simulink model "generic_src"  (Simulink 10.3)
settings: Solver=ode45  StartTime=0.0  StopTime=inf  RelTol=1e-3  EnableMultiTasking=on
undefined symbols (not defined in the file): Area_Front, Area_Rear, ay_max_off, ay_max_on, ay_per_mu_max_off, ay_per_mu_max_on, Brake_ratio, brake_valve_ctrl_kP, cat1mode1_higher, cat1mode1_lower, cat1mode2_higher, cat1mode2_lower, cat1mode3_higher, cat1mode3_lower, cat2mode1_higher, cat2mode1_lower, cat2mode2_higher, cat2mode2_lower, cat2mode3_higher, cat2mode3_lower, delta_vel, diff_lock_fac, diff_lock_off, diff_lock_on, ESP_ctrl_kD, ESP_ctrl_kI, ESP_ctrl_kP, ESP_ctrl_restore_kI, ESP_min_throttle_fac, f_ax, f_slip, g, higherlimit_highvel, higherlimit_lowvel, highervel_fac, highervelocity_fac, InitialConditionForIntegrator, limit_acc, limit_selectlow, limit_starting, limit_vdiff, locktime_throttle, lowerlimit_highvel, lowerlimit_lowvel, lowervel_fac, lowervelocity_fac, min_throttle, MPS2KMPH, MSR_ctrl_kD, MSR_ctrl_kI, MSR_ctrl_kP, MSR_min_throttle_fac, PID_kP_sideslip, PID_kP_yawrate, RADpS2RpM, rBrake, RpM2RADpS, SH_SL_switch, sideslip_vel_corr, sidesplip_deviation_max ... (+35)
libraries: CarMaker4SL x137, simulink x57, simulink_extras x6
(part 5 of 12)

== system generic_src/CarMaker/IPG Vehicle/PowerTrain/PTControl Example/PTC ClutchOut/CreateBus PTC ClutchOut2 ==
  In : Inport
  BusCreator : BusCreator  Inputs=3
  Demux : Demux  Outputs=3
      settings: DisplayOption=none
  Out : Outport  VectorParamsAs1DForOutWhenUnconnected=off
  wires:
  Demux/3 -> BusCreator/3  "PTC ClutchOut2 Trq_out_trg"
  Demux/2 -> BusCreator/2  "PTC ClutchOut2 rotv_out_trg"
  Demux/1 -> BusCreator/1  "PTC ClutchOut2 Pos"
  BusCreator/1 -> Out/1
  In/1 -> Demux/1

== system generic_src/CarMaker/IPG Vehicle/PowerTrain/PTControl Example/PTC ClutchOut/CreateBus PTC ClutchOut3 ==
  In : Inport
  BusCreator : BusCreator  Inputs=3
  Demux : Demux  Outputs=3
      settings: DisplayOption=none
  Out : Outport  VectorParamsAs1DForOutWhenUnconnected=off
  wires:
  Demux/3 -> BusCreator/3  "PTC ClutchOut3 Trq_out_trg"
  Demux/2 -> BusCreator/2  "PTC ClutchOut3 rotv_out_trg"
  Demux/1 -> BusCreator/1  "PTC ClutchOut3 Pos"
  BusCreator/1 -> Out/1
  In/1 -> Demux/1

== system generic_src/CarMaker/IPG Vehicle/PowerTrain/PTControl Example/PTC ClutchOut/CreateBus PTC ClutchOut4 ==
  In : Inport
  BusCreator : BusCreator  Inputs=3
  Demux : Demux  Outputs=3
      settings: DisplayOption=none
  Out : Outport  VectorParamsAs1DForOutWhenUnconnected=off
  wires:
  Demux/3 -> BusCreator/3  "PTC ClutchOut4 Trq_out_trg"
  Demux/2 -> BusCreator/2  "PTC ClutchOut4 rotv_out_trg"
  Demux/1 -> BusCreator/1  "PTC ClutchOut4 Pos"
  BusCreator/1 -> Out/1
  In/1 -> Demux/1

== system generic_src/CarMaker/IPG Vehicle/PowerTrain/PTControl Example/PTC ClutchOut/CreateBus PTC ClutchOut5 ==
  In : Inport
  BusCreator : BusCreator  Inputs=3
  Demux : Demux  Outputs=3
      settings: DisplayOption=none
  Out : Outport  VectorParamsAs1DForOutWhenUnconnected=off
  wires:
  Demux/3 -> BusCreator/3  "PTC ClutchOut5 Trq_out_trg"
  Demux/2 -> BusCreator/2  "PTC ClutchOut5 rotv_out_trg"
  Demux/1 -> BusCreator/1  "PTC ClutchOut5 Pos"
  BusCreator/1 -> Out/1
  In/1 -> Demux/1

== system generic_src/CarMaker/IPG Vehicle/PowerTrain/PTControl Example/PTC ClutchOut/CreateBus PTC ClutchOut6 ==
  In : Inport
  BusCreator : BusCreator  Inputs=3
  Demux : Demux  Outputs=3
      settings: DisplayOption=none
  Out : Outport  VectorParamsAs1DForOutWhenUnconnected=off
  wires:
  Demux/3 -> BusCreator/3  "PTC ClutchOut6 Trq_out_trg"
  Demux/2 -> BusCreator/2  "PTC ClutchOut6 rotv_out_trg"
  Demux/1 -> BusCreator/1  "PTC ClutchOut6 Pos"
  BusCreator/1 -> Out/1
  In/1 -> Demux/1

== system generic_src/CarMaker/IPG Vehicle/PowerTrain/PTControl Example/PTC ClutchOut/CreateBus PTC ClutchOut7 ==
  In : Inport
  BusCreator : BusCreator  Inputs=3
  Demux : Demux  Outputs=3
      settings: DisplayOption=none
  Out : Outport  VectorParamsAs1DForOutWhenUnconnected=off
  wires:
  Demux/3 -> BusCreator/3  "PTC ClutchOut7 Trq_out_trg"
  Demux/2 -> BusCreator/2  "PTC ClutchOut7 rotv_out_trg"
  Demux/1 -> BusCreator/1  "PTC ClutchOut7 Pos"
  BusCreator/1 -> Out/1
  In/1 -> Demux/1

== system generic_src/CarMaker/IPG Vehicle/PowerTrain/PTControl Example/PTC ClutchOut/CreateBus PTC ClutchOut8 ==
  In : Inport
  BusCreator : BusCreator  Inputs=3
  Demux : Demux  Outputs=3
      settings: DisplayOption=none
  Out : Outport  VectorParamsAs1DForOutWhenUnconnected=off
  wires:
  Demux/3 -> BusCreator/3  "PTC ClutchOut8 Trq_out_trg"
  Demux/2 -> BusCreator/2  "PTC ClutchOut8 rotv_out_trg"
  Demux/1 -> BusCreator/1  "PTC ClutchOut8 Pos"
  BusCreator/1 -> Out/1
  In/1 -> Demux/1

== system generic_src/CarMaker/IPG Vehicle/PowerTrain/PTControl Example/PTC ClutchOut/CreateBus PTC ClutchOut9 ==
  In : Inport
  BusCreator : BusCreator  Inputs=3
  Demux : Demux  Outputs=3
      settings: DisplayOption=none
  Out : Outport  VectorParamsAs1DForOutWhenUnconnected=off
  wires:
  Demux/3 -> BusCreator/3  "PTC ClutchOut9 Trq_out_trg"
  Demux/2 -> BusCreator/2  "PTC ClutchOut9 rotv_out_trg"
  Demux/1 -> BusCreator/1  "PTC ClutchOut9 Pos"
  BusCreator/1 -> Out/1
  In/1 -> Demux/1

== system generic_src/CarMaker/IPG Vehicle/PowerTrain/PTControl Example/PTC GearBoxOut/CreateBus PTC GearboxOut0 ==
  In : Inport
  BusCreator : BusCreator  Inputs=12
  Demux : Demux  Outputs=12
      settings: DisplayOption=none
  Out : Outport  VectorParamsAs1DForOutWhenUnconnected=off
  wires:
  Demux/12 -> BusCreator/12  "PTC GearboxOut0 Clutch_dis Trq_out_trg"
  Demux/11 -> BusCreator/11  "PTC GearboxOut0 Clutch_dis rotv_out_trg"
  Demux/10 -> BusCreator/10  "PTC GearboxOut0 Clutch_dis Pos"
  Demux/9 -> BusCreator/9  "PTC GearboxOut0 Clutch Trq_out_trg"
  Demux/8 -> BusCreator/8  "PTC GearboxOut0 Clutch rotv_out_trg"
  Demux/7 -> BusCreator/7  "PTC GearboxOut0 Clutch Pos"
  Demux/6 -> BusCreator/6  "PTC GearboxOut0 Trq_out_trg"
  Demux/5 -> BusCreator/5  "PTC GearboxOut0 rotv_in_trg"
  Demux/4 -> BusCreator/4  "PTC GearboxOut0 i_trg"
  Demux/3 -> BusCreator/3  "PTC GearboxOut0 set_ParkBrake"
  Demux/2 -> BusCreator/2  "PTC GearboxOut0 GearNoTrg_dis"
  Demux/1 -> BusCreator/1  "PTC GearboxOut0 GearNoTrg"
  BusCreator/1 -> Out/1
  In/1 -> Demux/1

== system generic_src/CarMaker/IPG Vehicle/PowerTrain/PTControl Example/PTC GearBoxOut/CreateBus PTC GearboxOut1 ==
  In : Inport
  BusCreator : BusCreator  Inputs=12
  Demux : Demux  Outputs=12
      settings: DisplayOption=none
  Out : Outport  VectorParamsAs1DForOutWhenUnconnected=off
  wires:
  Demux/12 -> BusCreator/12  "PTC GearboxOut1 Clutch_dis Trq_out_trg"
  Demux/11 -> BusCreator/11  "PTC GearboxOut1 Clutch_dis rotv_out_trg"
  Demux/10 -> BusCreator/10  "PTC GearboxOut1 Clutch_dis Pos"
  Demux/9 -> BusCreator/9  "PTC GearboxOut1 Clutch Trq_out_trg"
  Demux/8 -> BusCreator/8  "PTC GearboxOut1 Clutch rotv_out_trg"
  Demux/7 -> BusCreator/7  "PTC GearboxOut1 Clutch Pos"
  Demux/6 -> BusCreator/6  "PTC GearboxOut1 Trq_out_trg"
  Demux/5 -> BusCreator/5  "PTC GearboxOut1 rotv_in_trg"
  Demux/4 -> BusCreator/4  "PTC GearboxOut1 i_trg"
  Demux/3 -> BusCreator/3  "PTC GearboxOut1 set_ParkBrake"
  Demux/2 -> BusCreator/2  "PTC GearboxOut1 GearNoTrg_dis"
  Demux/1 -> BusCreator/1  "PTC GearboxOut1 GearNoTrg"
  BusCreator/1 -> Out/1
  In/1 -> Demux/1

== system generic_src/CarMaker/IPG Vehicle/PowerTrain/PTControl Example/PTC GearBoxOut/CreateBus PTC GearboxOut10 ==
  In : Inport
  BusCreator : BusCreator  Inputs=12
  Demux : Demux  Outputs=12
      settings: DisplayOption=none
  Out : Outport  VectorParamsAs1DForOutWhenUnconnected=off
  wires:
  Demux/12 -> BusCreator/12  "PTC GearboxOut10 Clutch_dis Trq_out_trg"
  Demux/11 -> BusCreator/11  "PTC GearboxOut10 Clutch_dis rotv_out_trg"
  Demux/10 -> BusCreator/10  "PTC GearboxOut10 Clutch_dis Pos"
  Demux/9 -> BusCreator/9  "PTC GearboxOut10 Clutch Trq_out_trg"
  Demux/8 -> BusCreator/8  "PTC GearboxOut10 Clutch rotv_out_trg"
  Demux/7 -> BusCreator/7  "PTC GearboxOut10 Clutch Pos"
  Demux/6 -> BusCreator/6  "PTC GearboxOut10 Trq_out_trg"
  Demux/5 -> BusCreator/5  "PTC GearboxOut10 rotv_in_trg"
  Demux/4 -> BusCreator/4  "PTC GearboxOut10 i_trg"
  Demux/3 -> BusCreator/3  "PTC GearboxOut10 set_ParkBrake"
  Demux/2 -> BusCreator/2  "PTC GearboxOut10 GearNoTrg_dis"
  Demux/1 -> BusCreator/1  "PTC GearboxOut10 GearNoTrg"
  BusCreator/1 -> Out/1
  In/1 -> Demux/1

== system generic_src/CarMaker/IPG Vehicle/PowerTrain/PTControl Example/PTC GearBoxOut/CreateBus PTC GearboxOut11 ==
  In : Inport
  BusCreator : BusCreator  Inputs=12
  Demux : Demux  Outputs=12
      settings: DisplayOption=none
  Out : Outport  VectorParamsAs1DForOutWhenUnconnected=off
  wires:
  Demux/12 -> BusCreator/12  "PTC GearboxOut11 Clutch_dis Trq_out_trg"
  Demux/11 -> BusCreator/11  "PTC GearboxOut11 Clutch_dis rotv_out_trg"
  Demux/10 -> BusCreator/10  "PTC GearboxOut11 Clutch_dis Pos"
  Demux/9 -> BusCreator/9  "PTC GearboxOut11 Clutch Trq_out_trg"
  Demux/8 -> BusCreator/8  "PTC GearboxOut11 Clutch rotv_out_trg"
  Demux/7 -> BusCreator/7  "PTC GearboxOut11 Clutch Pos"
  Demux/6 -> BusCreator/6  "PTC GearboxOut11 Trq_out_trg"
  Demux/5 -> BusCreator/5  "PTC GearboxOut11 rotv_in_trg"
  Demux/4 -> BusCreator/4  "PTC GearboxOut11 i_trg"
  Demux/3 -> BusCreator/3  "PTC GearboxOut11 set_ParkBrake"
  Demux/2 -> BusCreator/2  "PTC GearboxOut11 GearNoTrg_dis"
  Demux/1 -> BusCreator/1  "PTC GearboxOut11 GearNoTrg"
  BusCreator/1 -> Out/1
  In/1 -> Demux/1

== system generic_src/CarMaker/IPG Vehicle/PowerTrain/PTControl Example/PTC GearBoxOut/CreateBus PTC GearboxOut2 ==
  In : Inport
  BusCreator : BusCreator  Inputs=12
  Demux : Demux  Outputs=12
      settings: DisplayOption=none
  Out : Outport  VectorParamsAs1DForOutWhenUnconnected=off
  wires:
  Demux/12 -> BusCreator/12  "PTC GearboxOut2 Clutch_dis Trq_out_trg"
  Demux/11 -> BusCreator/11  "PTC GearboxOut2 Clutch_dis rotv_out_trg"
  Demux/10 -> BusCreator/10  "PTC GearboxOut2 Clutch_dis Pos"
  Demux/9 -> BusCreator/9  "PTC GearboxOut2 Clutch Trq_out_trg"
  Demux/8 -> BusCreator/8  "PTC GearboxOut2 Clutch rotv_out_trg"
  Demux/7 -> BusCreator/7  "PTC GearboxOut2 Clutch Pos"
  Demux/6 -> BusCreator/6  "PTC GearboxOut2 Trq_out_trg"
  Demux/5 -> BusCreator/5  "PTC GearboxOut2 rotv_in_trg"
  Demux/4 -> BusCreator/4  "PTC GearboxOut2 i_trg"
  Demux/3 -> BusCreator/3  "PTC GearboxOut2 set_ParkBrake"
  Demux/2 -> BusCreator/2  "PTC GearboxOut2 GearNoTrg_dis"
  Demux/1 -> BusCreator/1  "PTC GearboxOut2 GearNoTrg"
  BusCreator/1 -> Out/1
  In/1 -> Demux/1

== system generic_src/CarMaker/IPG Vehicle/PowerTrain/PTControl Example/PTC GearBoxOut/CreateBus PTC GearboxOut3 ==
  In : Inport
  BusCreator : BusCreator  Inputs=12
  Demux : Demux  Outputs=12
      settings: DisplayOption=none
  Out : Outport  VectorParamsAs1DForOutWhenUnconnected=off
  wires:
  Demux/12 -> BusCreator/12  "PTC GearboxOut3 Clutch_dis Trq_out_trg"
  Demux/11 -> BusCreator/11  "PTC GearboxOut3 Clutch_dis rotv_out_trg"
  Demux/10 -> BusCreator/10  "PTC GearboxOut3 Clutch_dis Pos"
  Demux/9 -> BusCreator/9  "PTC GearboxOut3 Clutch Trq_out_trg"
  Demux/8 -> BusCreator/8  "PTC GearboxOut3 Clutch rotv_out_trg"
  Demux/7 -> BusCreator/7  "PTC GearboxOut3 Clutch Pos"
  Demux/6 -> BusCreator/6  "PTC GearboxOut3 Trq_out_trg"
  Demux/5 -> BusCreator/5  "PTC GearboxOut3 rotv_in_trg"
  Demux/4 -> BusCreator/4  "PTC GearboxOut3 i_trg"
  Demux/3 -> BusCreator/3  "PTC GearboxOut3 set_ParkBrake"
  Demux/2 -> BusCreator/2  "PTC GearboxOut3 GearNoTrg_dis"
  Demux/1 -> BusCreator/1  "PTC GearboxOut3 GearNoTrg"
  BusCreator/1 -> Out/1
  In/1 -> Demux/1

== system generic_src/CarMaker/IPG Vehicle/PowerTrain/PTControl Example/PTC GearBoxOut/CreateBus PTC GearboxOut4 ==
  In : Inport
  BusCreator : BusCreator  Inputs=12
  Demux : Demux  Outputs=12
      settings: DisplayOption=none
  Out : Outport  VectorParamsAs1DForOutWhenUnconnected=off
  wires:
  Demux/12 -> BusCreator/12  "PTC GearboxOut4 Clutch_dis Trq_out_trg"
  Demux/11 -> BusCreator/11  "PTC GearboxOut4 Clutch_dis rotv_out_trg"
  Demux/10 -> BusCreator/10  "PTC GearboxOut4 Clutch_dis Pos"
  Demux/9 -> BusCreator/9  "PTC GearboxOut4 Clutch Trq_out_trg"
  Demux/8 -> BusCreator/8  "PTC GearboxOut4 Clutch rotv_out_trg"
  Demux/7 -> BusCreator/7  "PTC GearboxOut4 Clutch Pos"
  Demux/6 -> BusCreator/6  "PTC GearboxOut4 Trq_out_trg"
  Demux/5 -> BusCreator/5  "PTC GearboxOut4 rotv_in_trg"
  Demux/4 -> BusCreator/4  "PTC GearboxOut4 i_trg"
  Demux/3 -> BusCreator/3  "PTC GearboxOut4 set_ParkBrake"
  Demux/2 -> BusCreator/2  "PTC GearboxOut4 GearNoTrg_dis"
  Demux/1 -> BusCreator/1  "PTC GearboxOut4 GearNoTrg"
  BusCreator/1 -> Out/1
  In/1 -> Demux/1

== system generic_src/CarMaker/IPG Vehicle/PowerTrain/PTControl Example/PTC GearBoxOut/CreateBus PTC GearboxOut5 ==
  In : Inport
  BusCreator : BusCreator  Inputs=12
  Demux : Demux  Outputs=12
      settings: DisplayOption=none
  Out : Outport  VectorParamsAs1DForOutWhenUnconnected=off
  wires:
  Demux/12 -> BusCreator/12  "PTC GearboxOut5 Clutch_dis Trq_out_trg"
  Demux/11 -> BusCreator/11  "PTC GearboxOut5 Clutch_dis rotv_out_trg"
  Demux/10 -> BusCreator/10  "PTC GearboxOut5 Clutch_dis Pos"
  Demux/9 -> BusCreator/9  "PTC GearboxOut5 Clutch Trq_out_trg"
  Demux/8 -> BusCreator/8  "PTC GearboxOut5 Clutch rotv_out_trg"
  Demux/7 -> BusCreator/7  "PTC GearboxOut5 Clutch Pos"
  Demux/6 -> BusCreator/6  "PTC GearboxOut5 Trq_out_trg"
  Demux/5 -> BusCreator/5  "PTC GearboxOut5 rotv_in_trg"
  Demux/4 -> BusCreator/4  "PTC GearboxOut5 i_trg"
  Demux/3 -> BusCreator/3  "PTC GearboxOut5 set_ParkBrake"
  Demux/2 -> BusCreator/2  "PTC GearboxOut5 GearNoTrg_dis"
  Demux/1 -> BusCreator/1  "PTC GearboxOut5 GearNoTrg"
  BusCreator/1 -> Out/1
  In/1 -> Demux/1

== system generic_src/CarMaker/IPG Vehicle/PowerTrain/PTControl Example/PTC GearBoxOut/CreateBus PTC GearboxOut6 ==
  In : Inport
  BusCreator : BusCreator  Inputs=12
  Demux : Demux  Outputs=12
      settings: DisplayOption=none
  Out : Outport  VectorParamsAs1DForOutWhenUnconnected=off
  wires:
  Demux/12 -> BusCreator/12  "PTC GearboxOut6 Clutch_dis Trq_out_trg"
  Demux/11 -> BusCreator/11  "PTC GearboxOut6 Clutch_dis rotv_out_trg"
  Demux/10 -> BusCreator/10  "PTC GearboxOut6 Clutch_dis Pos"
  Demux/9 -> BusCreator/9  "PTC GearboxOut6 Clutch Trq_out_trg"
  Demux/8 -> BusCreator/8  "PTC GearboxOut6 Clutch rotv_out_trg"
  Demux/7 -> BusCreator/7  "PTC GearboxOut6 Clutch Pos"
  Demux/6 -> BusCreator/6  "PTC GearboxOut6 Trq_out_trg"
  Demux/5 -> BusCreator/5  "PTC GearboxOut6 rotv_in_trg"
  Demux/4 -> BusCreator/4  "PTC GearboxOut6 i_trg"
  Demux/3 -> BusCreator/3  "PTC GearboxOut6 set_ParkBrake"
  Demux/2 -> BusCreator/2  "PTC GearboxOut6 GearNoTrg_dis"
  Demux/1 -> BusCreator/1  "PTC GearboxOut6 GearNoTrg"
  BusCreator/1 -> Out/1
  In/1 -> Demux/1

== system generic_src/CarMaker/IPG Vehicle/PowerTrain/PTControl Example/PTC GearBoxOut/CreateBus PTC GearboxOut7 ==
  In : Inport
  BusCreator : BusCreator  Inputs=12
  Demux : Demux  Outputs=12
      settings: DisplayOption=none
  Out : Outport  VectorParamsAs1DForOutWhenUnconnected=off
  wires:
  Demux/12 -> BusCreator/12  "PTC GearboxOut7 Clutch_dis Trq_out_trg"
  Demux/11 -> BusCreator/11  "PTC GearboxOut7 Clutch_dis rotv_out_trg"
  Demux/10 -> BusCreator/10  "PTC GearboxOut7 Clutch_dis Pos"
  Demux/9 -> BusCreator/9  "PTC GearboxOut7 Clutch Trq_out_trg"
  Demux/8 -> BusCreator/8  "PTC GearboxOut7 Clutch rotv_out_trg"
  Demux/7 -> BusCreator/7  "PTC GearboxOut7 Clutch Pos"
  Demux/6 -> BusCreator/6  "PTC GearboxOut7 Trq_out_trg"
  Demux/5 -> BusCreator/5  "PTC GearboxOut7 rotv_in_trg"
  Demux/4 -> BusCreator/4  "PTC GearboxOut7 i_trg"
  Demux/3 -> BusCreator/3  "PTC GearboxOut7 set_ParkBrake"
  Demux/2 -> BusCreator/2  "PTC GearboxOut7 GearNoTrg_dis"
  Demux/1 -> BusCreator/1  "PTC GearboxOut7 GearNoTrg"
  BusCreator/1 -> Out/1
  In/1 -> Demux/1

== system generic_src/CarMaker/IPG Vehicle/PowerTrain/PTControl Example/PTC GearBoxOut/CreateBus PTC GearboxOut8 ==
  In : Inport
  BusCreator : BusCreator  Inputs=12
  Demux : Demux  Outputs=12
      settings: DisplayOption=none
  Out : Outport  VectorParamsAs1DForOutWhenUnconnected=off
  wires:
  Demux/12 -> BusCreator/12  "PTC GearboxOut8 Clutch_dis Trq_out_trg"
  Demux/11 -> BusCreator/11  "PTC GearboxOut8 Clutch_dis rotv_out_trg"
  Demux/10 -> BusCreator/10  "PTC GearboxOut8 Clutch_dis Pos"
  Demux/9 -> BusCreator/9  "PTC GearboxOut8 Clutch Trq_out_trg"
  Demux/8 -> BusCreator/8  "PTC GearboxOut8 Clutch rotv_out_trg"
  Demux/7 -> BusCreator/7  "PTC GearboxOut8 Clutch Pos"
  Demux/6 -> BusCreator/6  "PTC GearboxOut8 Trq_out_trg"
  Demux/5 -> BusCreator/5  "PTC GearboxOut8 rotv_in_trg"
  Demux/4 -> BusCreator/4  "PTC GearboxOut8 i_trg"
  Demux/3 -> BusCreator/3  "PTC GearboxOut8 set_ParkBrake"
  Demux/2 -> BusCreator/2  "PTC GearboxOut8 GearNoTrg_dis"
  Demux/1 -> BusCreator/1  "PTC GearboxOut8 GearNoTrg"
  BusCreator/1 -> Out/1
  In/1 -> Demux/1

== system generic_src/CarMaker/IPG Vehicle/PowerTrain/PTControl Example/PTC GearBoxOut/CreateBus PTC GearboxOut9 ==
  In : Inport
  BusCreator : BusCreator  Inputs=12
  Demux : Demux  Outputs=12
      settings: DisplayOption=none
  Out : Outport  VectorParamsAs1DForOutWhenUnconnected=off
  wires:
  Demux/12 -> BusCreator/12  "PTC GearboxOut9 Clutch_dis Trq_out_trg"
  Demux/11 -> BusCreator/11  "PTC GearboxOut9 Clutch_dis rotv_out_trg"
  Demux/10 -> BusCreator/10  "PTC GearboxOut9 Clutch_dis Pos"
  Demux/9 -> BusCreator/9  "PTC GearboxOut9 Clutch Trq_out_trg"
  Demux/8 -> BusCreator/8  "PTC GearboxOut9 Clutch rotv_out_trg"
  Demux/7 -> BusCreator/7  "PTC GearboxOut9 Clutch Pos"
  Demux/6 -> BusCreator/6  "PTC GearboxOut9 Trq_out_trg"
  Demux/5 -> BusCreator/5  "PTC GearboxOut9 rotv_in_trg"
  Demux/4 -> BusCreator/4  "PTC GearboxOut9 i_trg"
  Demux/3 -> BusCreator/3  "PTC GearboxOut9 set_ParkBrake"
  Demux/2 -> BusCreator/2  "PTC GearboxOut9 GearNoTrg_dis"
  Demux/1 -> BusCreator/1  "PTC GearboxOut9 GearNoTrg"
  BusCreator/1 -> Out/1
  In/1 -> Demux/1

== system generic_src/CarMaker/IPG Vehicle/PowerTrain/PTControl Example/PTC MotorOut/CreateBus PTC MotorOut0 ==
  In : Inport
  BusCreator : BusCreator  Inputs=3
  Demux : Demux  Outputs=3
      settings: DisplayOption=none
  Out : Outport  VectorParamsAs1DForOutWhenUnconnected=off
  wires:
  Demux/3 -> BusCreator/3  "PTC MotorOut0 rotv_trg"
  Demux/2 -> BusCreator/2  "PTC MotorOut0 Trq_trg"
  Demux/1 -> BusCreator/1  "PTC MotorOut0 Load"
  BusCreator/1 -> Out/1
  In/1 -> Demux/1

== system generic_src/CarMaker/IPG Vehicle/PowerTrain/PTControl Example/PTC MotorOut/CreateBus PTC MotorOut1 ==
  In : Inport
  BusCreator : BusCreator  Inputs=3
  Demux : Demux  Outputs=3
      settings: DisplayOption=none
  Out : Outport  VectorParamsAs1DForOutWhenUnconnected=off
  wires:
  Demux/3 -> BusCreator/3  "PTC MotorOut1 rotv_trg"
  Demux/2 -> BusCreator/2  "PTC MotorOut1 Trq_trg"
  Demux/1 -> BusCreator/1  "PTC MotorOut1 Load"
  BusCreator/1 -> Out/1
  In/1 -> Demux/1

== system generic_src/CarMaker/IPG Vehicle/PowerTrain/PTControl Example/PTC MotorOut/CreateBus PTC MotorOut10 ==
  In : Inport
  BusCreator : BusCreator  Inputs=3
  Demux : Demux  Outputs=3
      settings: DisplayOption=none
  Out : Outport  VectorParamsAs1DForOutWhenUnconnected=off
  wires:
  Demux/3 -> BusCreator/3  "PTC MotorOut10 rotv_trg"
  Demux/2 -> BusCreator/2  "PTC MotorOut10 Trq_trg"
  Demux/1 -> BusCreator/1  "PTC MotorOut10 Load"
  BusCreator/1 -> Out/1
  In/1 -> Demux/1

== system generic_src/CarMaker/IPG Vehicle/PowerTrain/PTControl Example/PTC MotorOut/CreateBus PTC MotorOut11 ==
  In : Inport
  BusCreator : BusCreator  Inputs=3
  Demux : Demux  Outputs=3
      settings: DisplayOption=none
  Out : Outport  VectorParamsAs1DForOutWhenUnconnected=off
  wires:
  Demux/3 -> BusCreator/3  "PTC MotorOut11 rotv_trg"
  Demux/2 -> BusCreator/2  "PTC MotorOut11 Trq_trg"
  Demux/1 -> BusCreator/1  "PTC MotorOut11 Load"
  BusCreator/1 -> Out/1
  In/1 -> Demux/1

== system generic_src/CarMaker/IPG Vehicle/PowerTrain/PTControl Example/PTC MotorOut/CreateBus PTC MotorOut2 ==
  In : Inport
  BusCreator : BusCreator  Inputs=3
  Demux : Demux  Outputs=3
      settings: DisplayOption=none
  Out : Outport  VectorParamsAs1DForOutWhenUnconnected=off
  wires:
  Demux/3 -> BusCreator/3  "PTC MotorOut2 rotv_trg"
  Demux/2 -> BusCreator/2  "PTC MotorOut2 Trq_trg"
  Demux/1 -> BusCreator/1  "PTC MotorOut2 Load"
  BusCreator/1 -> Out/1
  In/1 -> Demux/1

== system generic_src/CarMaker/IPG Vehicle/PowerTrain/PTControl Example/PTC MotorOut/CreateBus PTC MotorOut3 ==
  In : Inport
  BusCreator : BusCreator  Inputs=3
  Demux : Demux  Outputs=3
      settings: DisplayOption=none
  Out : Outport  VectorParamsAs1DForOutWhenUnconnected=off
  wires:
  Demux/3 -> BusCreator/3  "PTC MotorOut3 rotv_trg"
  Demux/2 -> BusCreator/2  "PTC MotorOut3 Trq_trg"
  Demux/1 -> BusCreator/1  "PTC MotorOut3 Load"
  BusCreator/1 -> Out/1
  In/1 -> Demux/1

== system generic_src/CarMaker/IPG Vehicle/PowerTrain/PTControl Example/PTC MotorOut/CreateBus PTC MotorOut4 ==
  In : Inport
  BusCreator : BusCreator  Inputs=3
  Demux : Demux  Outputs=3
      settings: DisplayOption=none
  Out : Outport  VectorParamsAs1DForOutWhenUnconnected=off
  wires:
  Demux/3 -> BusCreator/3  "PTC MotorOut4 rotv_trg"
  Demux/2 -> BusCreator/2  "PTC MotorOut4 Trq_trg"
  Demux/1 -> BusCreator/1  "PTC MotorOut4 Load"
  BusCreator/1 -> Out/1
  In/1 -> Demux/1

== system generic_src/CarMaker/IPG Vehicle/PowerTrain/PTControl Example/PTC MotorOut/CreateBus PTC MotorOut5 ==
  In : Inport
  BusCreator : BusCreator  Inputs=3
  Demux : Demux  Outputs=3
      settings: DisplayOption=none
  Out : Outport  VectorParamsAs1DForOutWhenUnconnected=off
  wires:
  Demux/3 -> BusCreator/3  "PTC MotorOut5 rotv_trg"
  Demux/2 -> BusCreator/2  "PTC MotorOut5 Trq_trg"
  Demux/1 -> BusCreator/1  "PTC MotorOut5 Load"
  BusCreator/1 -> Out/1
  In/1 -> Demux/1

== system generic_src/CarMaker/IPG Vehicle/PowerTrain/PTControl Example/PTC MotorOut/CreateBus PTC MotorOut6 ==
  In : Inport
  BusCreator : BusCreator  Inputs=3
  Demux : Demux  Outputs=3
      settings: DisplayOption=none
  Out : Outport  VectorParamsAs1DForOutWhenUnconnected=off
  wires:
  Demux/3 -> BusCreator/3  "PTC MotorOut6 rotv_trg"
  Demux/2 -> BusCreator/2  "PTC MotorOut6 Trq_trg"
  Demux/1 -> BusCreator/1  "PTC MotorOut6 Load"
  BusCreator/1 -> Out/1
  In/1 -> Demux/1

== system generic_src/CarMaker/IPG Vehicle/PowerTrain/PTControl Example/PTC MotorOut/CreateBus PTC MotorOut7 ==
  In : Inport
  BusCreator : BusCreator  Inputs=3
  Demux : Demux  Outputs=3
      settings: DisplayOption=none
  Out : Outport  VectorParamsAs1DForOutWhenUnconnected=off
  wires:
  Demux/3 -> BusCreator/3  "PTC MotorOut7 rotv_trg"
  Demux/2 -> BusCreator/2  "PTC MotorOut7 Trq_trg"
  Demux/1 -> BusCreator/1  "PTC MotorOut7 Load"
  BusCreator/1 -> Out/1
  In/1 -> Demux/1

== system generic_src/CarMaker/IPG Vehicle/PowerTrain/PTControl Example/PTC MotorOut/CreateBus PTC MotorOut8 ==
  In : Inport
  BusCreator : BusCreator  Inputs=3
  Demux : Demux  Outputs=3
      settings: DisplayOption=none
  Out : Outport  VectorParamsAs1DForOutWhenUnconnected=off
  wires:
  Demux/3 -> BusCreator/3  "PTC MotorOut8 rotv_trg"
  Demux/2 -> BusCreator/2  "PTC MotorOut8 Trq_trg"
  Demux/1 -> BusCreator/1  "PTC MotorOut8 Load"
  BusCreator/1 -> Out/1
  In/1 -> Demux/1

== system generic_src/CarMaker/IPG Vehicle/PowerTrain/PTControl Example/PTC MotorOut/CreateBus PTC MotorOut9 ==
  In : Inport
  BusCreator : BusCreator  Inputs=3
  Demux : Demux  Outputs=3
      settings: DisplayOption=none
  Out : Outport  VectorParamsAs1DForOutWhenUnconnected=off
  wires:
  Demux/3 -> BusCreator/3  "PTC MotorOut9 rotv_trg"
  Demux/2 -> BusCreator/2  "PTC MotorOut9 Trq_trg"
  Demux/1 -> BusCreator/1  "PTC MotorOut9 Load"
  BusCreator/1 -> Out/1
  In/1 -> Demux/1

== system generic_src/CarMaker/IPG Vehicle/PowerTrain/PTControl Example/PTControl Example/Engine ==
  Gas : Inport
  Engine_on : Inport  Port=2
  Constant : Constant
  Constant1 : Constant  Value=0
  Constant3 : Constant  Value=0
  Mux : Mux  Inputs=5
  NOTSET0 : Constant  Value=-99999
  NOTSET1 : Constant  Value=-99999
  NOTSET2 : Constant  Value=-99999
  Switch : Switch  Criteria=u2 ~= 0
  Switch1 : Switch  Criteria=u2 ~= 0
  EngineOut : Outport  VectorParamsAs1DForOutWhenUnconnected=off
  wires:
  Constant/1 -> Switch/1
  Mux/1 -> EngineOut/1
  Constant1/1 -> Switch/3
  Engine_on/1 -> Switch/2, Switch1/2
  Gas/1 -> Switch1/1
  Constant3/1 -> Switch1/3
  NOTSET1/1 -> Mux/5  "rotv_trg"
  NOTSET2/1 -> Mux/4  "Trq_trg"
  Switch1/1 -> Mux/3  "Load"
  NOTSET0/1 -> Mux/2  "FuelCutOff"
  Switch/1 -> Mux/1  "set_ISC"

== system generic_src/CarMaker/IPG Vehicle/PowerTrain/PTControl Example/PTControl Example/ISG ==
  Key : Inport
  Constant : Constant
  Constant1 : Constant  Value=0
  KeyPos_KeyIn_Starter : Constant  Value=4
  Mux : Mux  Inputs=3
  NOTSET : Constant  Value=-99999
  NOTSET1 : Constant  Value=-99999
  Relational Operator1 : RelationalOperator  Operator===  OutDataTypeStr=boolean  RndMeth=Nearest
  Switch : Switch  Criteria=u2 ~= 0
  ISGOut : Outport  VectorParamsAs1DForOutWhenUnconnected=off
  wires:
  KeyPos_KeyIn_Starter/1 -> Relational Operator1/2
  Constant/1 -> Switch/1
  Constant1/1 -> Switch/3
  Relational Operator1/1 -> Switch/2
  Key/1 -> Relational Operator1/1
  Switch/1 -> Mux/1  "Load"
  NOTSET/1 -> Mux/2  "Trq_trg"
  NOTSET1/1 -> Mux/3  "rotv_trg"
  Mux/1 -> ISGOut/1

== system generic_src/CarMaker/IPG Vehicle/PowerTrain/PTControl Example/PTControl Example/PTC ==
  Key : Inport
  Engine_on : Inport  Port=2
  Constant : Constant
  Constant1 : Constant  Value=0
  Ground : Ground
  KeyPos2OperState : Lookup  InputValues=[0 1 2 3 4 5 6 7 8 9]  Table=[0 1 2 3 3 3 3 3 3 3]
  KeyPos_KeyIn_PowerOn : Constant  Value=3
  Logical Operator : Logic  AllPortsSameDT=off  OutDataTypeStr=boolean
  Mode_EngineDrive : Constant  Value=8
  Mux : Mux
  OperState_Driving : Constant  Value=4
  OperState_PowerOn : Constant  Value=3
  Relational Operator : RelationalOperator  OutDataTypeStr=boolean  RndMeth=Nearest
  Relational Operator1 : RelationalOperator  OutDataTypeStr=boolean  RndMeth=Nearest
  Switch : Switch  Criteria=u2 ~= 0
  Switch1 : Switch  Criteria=u2 ~= 0
  PTC MiscOut : Outport  VectorParamsAs1DForOutWhenUnconnected=off
  wires:
  KeyPos_KeyIn_PowerOn/1 -> Relational Operator/2
  Ground/1 -> Mux/2  "OperationError"
  Mux/1 -> PTC MiscOut/1
  Key/1 -> KeyPos2OperState/1, Relational Operator/1
  Constant/1 -> Switch/1
  Constant1/1 -> Switch/3
  Relational Operator/1 -> Switch/2  "Ignition"
  OperState_Driving/1 -> Switch1/1
  Switch1/1 -> Mux/1  "OperationState"
  KeyPos2OperState/1 -> Relational Operator1/1, Switch1/3  "OperationState"
  Logical Operator/1 -> Switch1/2
  Engine_on/1 -> Logical Operator/1
  Relational Operator1/1 -> Logical Operator/2
  OperState_PowerOn/1 -> Relational Operator1/2
  Switch/1 -> Mux/4  "Ignition"
  Mode_EngineDrive/1 -> Mux/3

== system generic_src/CarMaker/IPG Vehicle/PowerTrain/PTControl Example/PTControl_In/CreateBus PTC BatteryHVIn ==
  In : Inport
  BusCreator : BusCreator  Inputs=8
  Demux : Demux  Outputs=8
      settings: DisplayOption=none
  Out : Outport  VectorParamsAs1DForOutWhenUnconnected=off
  wires:
  Demux/5 -> BusCreator/5  "PTC BattHVIn Energy"
  Demux/4 -> BusCreator/4  "PTC BattHVIn AOC"
  BusCreator/1 -> Out/1
  Demux/2 -> BusCreator/2  "PTC BattHVIn SOH"
  Demux/3 -> BusCreator/3  "PTC BattHVIn Current"
  Demux/1 -> BusCreator/1  "PTC BattHVIn SOC"
  Demux/6 -> BusCreator/6  "PTC BattHVIn Pwr_max"
  Demux/8 -> BusCreator/8  "PTC BattHVIn TempCool_out"
  In/1 -> Demux/1
  Demux/7 -> BusCreator/7  "PTC BattHVIn Temp"

== system generic_src/CarMaker/IPG Vehicle/PowerTrain/PTControl Example/PTControl_In/CreateBus PTC BatteryLVIn ==
  In : Inport
  BusCreator : BusCreator  Inputs=8
  Demux : Demux  Outputs=8
      settings: DisplayOption=none
  Out : Outport  VectorParamsAs1DForOutWhenUnconnected=off
  wires:
  Demux/7 -> BusCreator/7  "PTC BattLVIn Temp"
  In/1 -> Demux/1
  Demux/8 -> BusCreator/8  "PTC BattLVIn TempCool_out"
  Demux/6 -> BusCreator/6  "PTC BattLVIn Pwr_max"
  Demux/1 -> BusCreator/1  "PTC BattLVIn SOC"
  Demux/3 -> BusCreator/3  "PTC BattLVIn Current"
  Demux/2 -> BusCreator/2  "PTC BattLVIn SOH"
  BusCreator/1 -> Out/1
  Demux/4 -> BusCreator/4  "PTC BattLVIn AOC"
  Demux/5 -> BusCreator/5  "PTC BattLVIn Energy"

== system generic_src/CarMaker/IPG Vehicle/PowerTrain/PTControl Example/PTControl_In/CreateBus PTC ClutchIn0 ==
  In : Inport
  BusCreator : BusCreator  Inputs=6
  Demux : Demux  Outputs=6
      settings: DisplayOption=none
  Out : Outport  VectorParamsAs1DForOutWhenUnconnected=off
  wires:
  Demux/6 -> BusCreator/6  "PTC ClutchIn0 i_TrqIn2Out"
  Demux/5 -> BusCreator/5  "PTC ClutchIn0 Trq_out"
  Demux/4 -> BusCreator/4  "PTC ClutchIn0 Trq_in"
  Demux/3 -> BusCreator/3  "PTC ClutchIn0 rotv_out"
  Demux/2 -> BusCreator/2  "PTC ClutchIn0 rotv_in"
  Demux/1 -> BusCreator/1  "PTC ClutchIn0 Pos"
  BusCreator/1 -> Out/1
  In/1 -> Demux/1

== system generic_src/CarMaker/IPG Vehicle/PowerTrain/PTControl Example/PTControl_In/CreateBus PTC ClutchIn1 ==
  In : Inport
  BusCreator : BusCreator  Inputs=6
  Demux : Demux  Outputs=6
      settings: DisplayOption=none
  Out : Outport  VectorParamsAs1DForOutWhenUnconnected=off
  wires:
  Demux/6 -> BusCreator/6  "PTC ClutchIn1 i_TrqIn2Out"
  Demux/5 -> BusCreator/5  "PTC ClutchIn1 Trq_out"
  Demux/4 -> BusCreator/4  "PTC ClutchIn1 Trq_in"
  Demux/3 -> BusCreator/3  "PTC ClutchIn1 rotv_out"
  Demux/2 -> BusCreator/2  "PTC ClutchIn1 rotv_in"
  Demux/1 -> BusCreator/1  "PTC ClutchIn1 Pos"
  BusCreator/1 -> Out/1
  In/1 -> Demux/1

== system generic_src/CarMaker/IPG Vehicle/PowerTrain/PTControl Example/PTControl_In/CreateBus PTC ClutchIn10 ==
  In : Inport
  BusCreator : BusCreator  Inputs=6
  Demux : Demux  Outputs=6
      settings: DisplayOption=none
  Out : Outport  VectorParamsAs1DForOutWhenUnconnected=off
  wires:
  Demux/6 -> BusCreator/6  "PTC ClutchIn10 i_TrqIn2Out"
  Demux/5 -> BusCreator/5  "PTC ClutchIn10 Trq_out"
  Demux/4 -> BusCreator/4  "PTC ClutchIn10 Trq_in"
  Demux/3 -> BusCreator/3  "PTC ClutchIn10 rotv_out"
  Demux/2 -> BusCreator/2  "PTC ClutchIn10 rotv_in"
  Demux/1 -> BusCreator/1  "PTC ClutchIn10 Pos"
  BusCreator/1 -> Out/1
  In/1 -> Demux/1

== system generic_src/CarMaker/IPG Vehicle/PowerTrain/PTControl Example/PTControl_In/CreateBus PTC ClutchIn11 ==
  In : Inport
  BusCreator : BusCreator  Inputs=6
  Demux : Demux  Outputs=6
      settings: DisplayOption=none
  Out : Outport  VectorParamsAs1DForOutWhenUnconnected=off
  wires:
  Demux/6 -> BusCreator/6  "PTC ClutchIn11 i_TrqIn2Out"
  Demux/5 -> BusCreator/5  "PTC ClutchIn11 Trq_out"
  Demux/4 -> BusCreator/4  "PTC ClutchIn11 Trq_in"
  Demux/3 -> BusCreator/3  "PTC ClutchIn11 rotv_out"
  Demux/2 -> BusCreator/2  "PTC ClutchIn11 rotv_in"
  Demux/1 -> BusCreator/1  "PTC ClutchIn11 Pos"
  BusCreator/1 -> Out/1
  In/1 -> Demux/1

== system generic_src/CarMaker/IPG Vehicle/PowerTrain/PTControl Example/PTControl_In/CreateBus PTC ClutchIn2 ==
  In : Inport
  BusCreator : BusCreator  Inputs=6
  Demux : Demux  Outputs=6
      settings: DisplayOption=none
  Out : Outport  VectorParamsAs1DForOutWhenUnconnected=off
  wires:
  Demux/6 -> BusCreator/6  "PTC ClutchIn2 i_TrqIn2Out"
  Demux/5 -> BusCreator/5  "PTC ClutchIn2 Trq_out"
  Demux/4 -> BusCreator/4  "PTC ClutchIn2 Trq_in"
  Demux/3 -> BusCreator/3  "PTC ClutchIn2 rotv_out"
  Demux/2 -> BusCreator/2  "PTC ClutchIn2 rotv_in"
  Demux/1 -> BusCreator/1  "PTC ClutchIn2 Pos"
  BusCreator/1 -> Out/1
  In/1 -> Demux/1

== system generic_src/CarMaker/IPG Vehicle/PowerTrain/PTControl Example/PTControl_In/CreateBus PTC ClutchIn3 ==
  In : Inport
  BusCreator : BusCreator  Inputs=6
  Demux : Demux  Outputs=6
      settings: DisplayOption=none
  Out : Outport  VectorParamsAs1DForOutWhenUnconnected=off
  wires:
  Demux/6 -> BusCreator/6  "PTC ClutchIn3 i_TrqIn2Out"
  Demux/5 -> BusCreator/5  "PTC ClutchIn3 Trq_out"
  Demux/4 -> BusCreator/4  "PTC ClutchIn3 Trq_in"
  Demux/3 -> BusCreator/3  "PTC ClutchIn3 rotv_out"
  Demux/2 -> BusCreator/2  "PTC ClutchIn3 rotv_in"
  Demux/1 -> BusCreator/1  "PTC ClutchIn3 Pos"
  BusCreator/1 -> Out/1
  In/1 -> Demux/1

== system generic_src/CarMaker/IPG Vehicle/PowerTrain/PTControl Example/PTControl_In/CreateBus PTC ClutchIn4 ==
  In : Inport
  BusCreator : BusCreator  Inputs=6
  Demux : Demux  Outputs=6
      settings: DisplayOption=none
  Out : Outport  VectorParamsAs1DForOutWhenUnconnected=off
  wires:
  Demux/6 -> BusCreator/6  "PTC ClutchIn4 i_TrqIn2Out"
  Demux/5 -> BusCreator/5  "PTC ClutchIn4 Trq_out"
  Demux/4 -> BusCreator/4  "PTC ClutchIn4 Trq_in"
  Demux/3 -> BusCreator/3  "PTC ClutchIn4 rotv_out"
  Demux/2 -> BusCreator/2  "PTC ClutchIn4 rotv_in"
  Demux/1 -> BusCreator/1  "PTC ClutchIn4 Pos"
  BusCreator/1 -> Out/1
  In/1 -> Demux/1

== system generic_src/CarMaker/IPG Vehicle/PowerTrain/PTControl Example/PTControl_In/CreateBus PTC ClutchIn5 ==
  In : Inport
  BusCreator : BusCreator  Inputs=6
  Demux : Demux  Outputs=6
      settings: DisplayOption=none
  Out : Outport  VectorParamsAs1DForOutWhenUnconnected=off
  wires:
  Demux/6 -> BusCreator/6  "PTC ClutchIn5 i_TrqIn2Out"
  Demux/5 -> BusCreator/5  "PTC ClutchIn5 Trq_out"
  Demux/4 -> BusCreator/4  "PTC ClutchIn5 Trq_in"
  Demux/3 -> BusCreator/3  "PTC ClutchIn5 rotv_out"
  Demux/2 -> BusCreator/2  "PTC ClutchIn5 rotv_in"
  Demux/1 -> BusCreator/1  "PTC ClutchIn5 Pos"
  BusCreator/1 -> Out/1
  In/1 -> Demux/1

== system generic_src/CarMaker/IPG Vehicle/PowerTrain/PTControl Example/PTControl_In/CreateBus PTC ClutchIn6 ==
  In : Inport
  BusCreator : BusCreator  Inputs=6
  Demux : Demux  Outputs=6
      settings: DisplayOption=none
  Out : Outport  VectorParamsAs1DForOutWhenUnconnected=off
  wires:
  Demux/6 -> BusCreator/6  "PTC ClutchIn6 i_TrqIn2Out"
  Demux/5 -> BusCreator/5  "PTC ClutchIn6 Trq_out"
  Demux/4 -> BusCreator/4  "PTC ClutchIn6 Trq_in"
  Demux/3 -> BusCreator/3  "PTC ClutchIn6 rotv_out"
  Demux/2 -> BusCreator/2  "PTC ClutchIn6 rotv_in"
  Demux/1 -> BusCreator/1  "PTC ClutchIn6 Pos"
  BusCreator/1 -> Out/1
  In/1 -> Demux/1

== system generic_src/CarMaker/IPG Vehicle/PowerTrain/PTControl Example/PTControl_In/CreateBus PTC ClutchIn7 ==
  In : Inport
  BusCreator : BusCreator  Inputs=6
  Demux : Demux  Outputs=6
      settings: DisplayOption=none
  Out : Outport  VectorParamsAs1DForOutWhenUnconnected=off
  wires:
  Demux/6 -> BusCreator/6  "PTC ClutchIn7 i_TrqIn2Out"
  Demux/5 -> BusCreator/5  "PTC ClutchIn7 Trq_out"
  Demux/4 -> BusCreator/4  "PTC ClutchIn7 Trq_in"
  Demux/3 -> BusCreator/3  "PTC ClutchIn7 rotv_out"
  Demux/2 -> BusCreator/2  "PTC ClutchIn7 rotv_in"
  Demux/1 -> BusCreator/1  "PTC ClutchIn7 Pos"
  BusCreator/1 -> Out/1
  In/1 -> Demux/1

== system generic_src/CarMaker/IPG Vehicle/PowerTrain/PTControl Example/PTControl_In/CreateBus PTC ClutchIn8 ==
  In : Inport
  BusCreator : BusCreator  Inputs=6
  Demux : Demux  Outputs=6
      settings: DisplayOption=none
  Out : Outport  VectorParamsAs1DForOutWhenUnconnected=off
  wires:
  Demux/6 -> BusCreator/6  "PTC ClutchIn8 i_TrqIn2Out"
  Demux/5 -> BusCreator/5  "PTC ClutchIn8 Trq_out"
  Demux/4 -> BusCreator/4  "PTC ClutchIn8 Trq_in"
  Demux/3 -> BusCreator/3  "PTC ClutchIn8 rotv_out"
  Demux/2 -> BusCreator/2  "PTC ClutchIn8 rotv_in"
  Demux/1 -> BusCreator/1  "PTC ClutchIn8 Pos"
  BusCreator/1 -> Out/1
  In/1 -> Demux/1

== system generic_src/CarMaker/IPG Vehicle/PowerTrain/PTControl Example/PTControl_In/CreateBus PTC ClutchIn9 ==
  In : Inport
  BusCreator : BusCreator  Inputs=6
  Demux : Demux  Outputs=6
      settings: DisplayOption=none
  Out : Outport  VectorParamsAs1DForOutWhenUnconnected=off
  wires:
  Demux/6 -> BusCreator/6  "PTC ClutchIn9 i_TrqIn2Out"
  Demux/5 -> BusCreator/5  "PTC ClutchIn9 Trq_out"
  Demux/4 -> BusCreator/4  "PTC ClutchIn9 Trq_in"
  Demux/3 -> BusCreator/3  "PTC ClutchIn9 rotv_out"
  Demux/2 -> BusCreator/2  "PTC ClutchIn9 rotv_in"
  Demux/1 -> BusCreator/1  "PTC ClutchIn9 Pos"
  BusCreator/1 -> Out/1
  In/1 -> Demux/1

== system generic_src/CarMaker/IPG Vehicle/PowerTrain/PTControl Example/PTControl_In/CreateBus PTC Control Units ==
  In : Inport
  BusCreator : BusCreator  Inputs=4
  Demux : Demux
      settings: DisplayOption=none
  Out : Outport  VectorParamsAs1DForOutWhenUnconnected=off
  wires:
  Demux/4 -> BusCreator/4  "PTC BCU_Status"
  Demux/3 -> BusCreator/3  "PTC TCU_Status"
  Demux/2 -> BusCreator/2  "PTC MCU_Status"
  Demux/1 -> BusCreator/1  "PTC ECU_Status"
  BusCreator/1 -> Out/1
  In/1 -> Demux/1

== system generic_src/CarMaker/IPG Vehicle/PowerTrain/PTControl Example/PTControl_In/CreateBus PTC DriveSrcIn ==
  In : Inport
  BusCreator : BusCreator  Inputs=4
  Demux : Demux
      settings: DisplayOption=none
  Out : Outport  VectorParamsAs1DForOutWhenUnconnected=off
  wires:
  Demux/4 -> BusCreator/4  "PTC DriveSrcIn_d3 Trq_DriveSrc_trg"
  Demux/3 -> BusCreator/3  "PTC DriveSrcIn_d2 Trq_DriveSrc_trg"
  Demux/2 -> BusCreator/2  "PTC DriveSrcIn_d1 Trq_DriveSrc_trg"
  Demux/1 -> BusCreator/1  "PTC DriveSrcIn_d0 Trq_DriveSrc_trg"
  BusCreator/1 -> Out/1
  In/1 -> Demux/1

== system generic_src/CarMaker/IPG Vehicle/PowerTrain/PTControl Example/PTControl_In/CreateBus PTC EngineIn ==
  In : Inport
  BusCreator : BusCreator  Inputs=7
  Demux : Demux  Outputs=7
      settings: DisplayOption=none
  Out : Outport  VectorParamsAs1DForOutWhenUnconnected=off
  wires:
  Demux/7 -> BusCreator/7  "PTC EngineIn FuelFlow"
  Demux/6 -> BusCreator/6  "PTC EngineIn TrqOpt"
  Demux/5 -> BusCreator/5  "PTC EngineIn TrqFull"
  Demux/4 -> BusCreator/4  "PTC EngineIn TrqDrag"
  Demux/3 -> BusCreator/3  "PTC EngineIn Trq"
  Demux/2 -> BusCreator/2  "PTC EngineIn rotv"
  Demux/1 -> BusCreator/1  "PTC EngineIn Engine_on"
  BusCreator/1 -> Out/1
  In/1 -> Demux/1

== system generic_src/CarMaker/IPG Vehicle/PowerTrain/PTControl Example/PTControl_In/CreateBus PTC GearboxIn0 ==
  In : Inport
  BusCreator : BusCreator  Inputs=20
  Demux : Demux  Outputs=20
      settings: DisplayOption=none
  Out : Outport  VectorParamsAs1DForOutWhenUnconnected=off
  wires:
  Demux/20 -> BusCreator/20  "PTC GearboxIn0 Clutch_dis i_TrqIn2Out"
  Demux/19 -> BusCreator/19  "PTC GearboxIn0 Clutch_dis Trq_out"
  Demux/18 -> BusCreator/18  "PTC GearboxIn0 Clutch_dis Trq_in"
  Demux/17 -> BusCreator/17  "PTC GearboxIn0 Clutch_dis rotv_out"
  Demux/16 -> BusCreator/16  "PTC GearboxIn0 Clutch_dis rotv_in"
  Demux/15 -> BusCreator/15  "PTC GearboxIn0 Clutch_dis Pos"
  Demux/14 -> BusCreator/14  "PTC GearboxIn0 Clutch i_TrqIn2Out"
  Demux/13 -> BusCreator/13  "PTC GearboxIn0 Clutch Trq_out"
  Demux/12 -> BusCreator/12  "PTC GearboxIn0 Clutch Trq_in"
  Demux/11 -> BusCreator/11  "PTC GearboxIn0 Clutch rotv_out"
  Demux/10 -> BusCreator/10  "PTC GearboxIn0 Clutch rotv_in"
  Demux/9 -> BusCreator/9  "PTC GearboxIn0 Clutch Pos"
  Demux/8 -> BusCreator/8  "PTC GearboxIn0 Trq_out"
  Demux/7 -> BusCreator/7  "PTC GearboxIn0 Trq_in"
  Demux/6 -> BusCreator/6  "PTC GearboxIn0 rotv_out"
  Demux/5 -> BusCreator/5  "PTC GearboxIn0 rotv_in"
  Demux/4 -> BusCreator/4  "PTC GearboxIn0 i"
  Demux/3 -> BusCreator/3  "PTC GearboxIn0 Trq_DriveSrc_trg"
  Demux/2 -> BusCreator/2  "PTC GearboxIn0 GearNo_dis"
  Demux/1 -> BusCreator/1  "PTC GearboxIn0 GearNo"
  BusCreator/1 -> Out/1
  In/1 -> Demux/1

== system generic_src/CarMaker/IPG Vehicle/PowerTrain/PTControl Example/PTControl_In/CreateBus PTC GearboxIn1 ==
  In : Inport
  BusCreator : BusCreator  Inputs=20
  Demux : Demux  Outputs=20
      settings: DisplayOption=none
  Out : Outport  VectorParamsAs1DForOutWhenUnconnected=off
  wires:
  Demux/20 -> BusCreator/20  "PTC GearboxIn1 Clutch_dis i_TrqIn2Out"
  Demux/19 -> BusCreator/19  "PTC GearboxIn1 Clutch_dis Trq_out"
  Demux/18 -> BusCreator/18  "PTC GearboxIn1 Clutch_dis Trq_in"
  Demux/17 -> BusCreator/17  "PTC GearboxIn1 Clutch_dis rotv_out"
  Demux/16 -> BusCreator/16  "PTC GearboxIn1 Clutch_dis rotv_in"
  Demux/15 -> BusCreator/15  "PTC GearboxIn1 Clutch_dis Pos"
  Demux/14 -> BusCreator/14  "PTC GearboxIn1 Clutch i_TrqIn2Out"
  Demux/13 -> BusCreator/13  "PTC GearboxIn1 Clutch Trq_out"
  Demux/12 -> BusCreator/12  "PTC GearboxIn1 Clutch Trq_in"
  Demux/11 -> BusCreator/11  "PTC GearboxIn1 Clutch rotv_out"
  Demux/10 -> BusCreator/10  "PTC GearboxIn1 Clutch rotv_in"
  Demux/9 -> BusCreator/9  "PTC GearboxIn1 Clutch Pos"
  Demux/8 -> BusCreator/8  "PTC GearboxIn1 Trq_out"
  Demux/7 -> BusCreator/7  "PTC GearboxIn1 Trq_in"
  Demux/6 -> BusCreator/6  "PTC GearboxIn1 rotv_out"
  Demux/5 -> BusCreator/5  "PTC GearboxIn1 rotv_in"
  Demux/4 -> BusCreator/4  "PTC GearboxIn1 i"
  Demux/3 -> BusCreator/3  "PTC GearboxIn1 Trq_DriveSrc_trg"
  Demux/2 -> BusCreator/2  "PTC GearboxIn1 GearNo_dis"
  Demux/1 -> BusCreator/1  "PTC GearboxIn1 GearNo"
  BusCreator/1 -> Out/1
  In/1 -> Demux/1

== system generic_src/CarMaker/IPG Vehicle/PowerTrain/PTControl Example/PTControl_In/CreateBus PTC GearboxIn10 ==
  In : Inport
  BusCreator : BusCreator  Inputs=20
  Demux : Demux  Outputs=20
      settings: DisplayOption=none
  Out : Outport  VectorParamsAs1DForOutWhenUnconnected=off
  wires:
  Demux/20 -> BusCreator/20  "PTC GearboxIn10 Clutch_dis i_TrqIn2Out"
  Demux/19 -> BusCreator/19  "PTC GearboxIn10 Clutch_dis Trq_out"
  Demux/18 -> BusCreator/18  "PTC GearboxIn10 Clutch_dis Trq_in"
  Demux/17 -> BusCreator/17  "PTC GearboxIn10 Clutch_dis rotv_out"
  Demux/16 -> BusCreator/16  "PTC GearboxIn10 Clutch_dis rotv_in"
  Demux/15 -> BusCreator/15  "PTC GearboxIn10 Clutch_dis Pos"
  Demux/14 -> BusCreator/14  "PTC GearboxIn10 Clutch i_TrqIn2Out"
  Demux/13 -> BusCreator/13  "PTC GearboxIn10 Clutch Trq_out"
  Demux/12 -> BusCreator/12  "PTC GearboxIn10 Clutch Trq_in"
  Demux/11 -> BusCreator/11  "PTC GearboxIn10 Clutch rotv_out"
  Demux/10 -> BusCreator/10  "PTC GearboxIn10 Clutch rotv_in"
  Demux/9 -> BusCreator/9  "PTC GearboxIn10 Clutch Pos"
  Demux/8 -> BusCreator/8  "PTC GearboxIn10 Trq_out"
  Demux/7 -> BusCreator/7  "PTC GearboxIn10 Trq_in"
  Demux/6 -> BusCreator/6  "PTC GearboxIn10 rotv_out"
  Demux/5 -> BusCreator/5  "PTC GearboxIn10 rotv_in"
  Demux/4 -> BusCreator/4  "PTC GearboxIn10 i"
  Demux/3 -> BusCreator/3  "PTC GearboxIn10 Trq_DriveSrc_trg"
  Demux/2 -> BusCreator/2  "PTC GearboxIn10 GearNo_dis"
  Demux/1 -> BusCreator/1  "PTC GearboxIn10 GearNo"
  BusCreator/1 -> Out/1
  In/1 -> Demux/1

== system generic_src/CarMaker/IPG Vehicle/PowerTrain/PTControl Example/PTControl_In/CreateBus PTC GearboxIn11 ==
  In : Inport
  BusCreator : BusCreator  Inputs=20
  Demux : Demux  Outputs=20
      settings: DisplayOption=none
  Out : Outport  VectorParamsAs1DForOutWhenUnconnected=off
  wires:
  Demux/20 -> BusCreator/20  "PTC GearboxIn11 Clutch_dis i_TrqIn2Out"
  Demux/19 -> BusCreator/19  "PTC GearboxIn11 Clutch_dis Trq_out"
  Demux/18 -> BusCreator/18  "PTC GearboxIn11 Clutch_dis Trq_in"
  Demux/17 -> BusCreator/17  "PTC GearboxIn11 Clutch_dis rotv_out"
  Demux/16 -> BusCreator/16  "PTC GearboxIn11 Clutch_dis rotv_in"
  Demux/15 -> BusCreator/15  "PTC GearboxIn11 Clutch_dis Pos"
  Demux/14 -> BusCreator/14  "PTC GearboxIn11 Clutch i_TrqIn2Out"
  Demux/13 -> BusCreator/13  "PTC GearboxIn11 Clutch Trq_out"
  Demux/12 -> BusCreator/12  "PTC GearboxIn11 Clutch Trq_in"
  Demux/11 -> BusCreator/11  "PTC GearboxIn11 Clutch rotv_out"
  Demux/10 -> BusCreator/10  "PTC GearboxIn11 Clutch rotv_in"
  Demux/9 -> BusCreator/9  "PTC GearboxIn11 Clutch Pos"
  Demux/8 -> BusCreator/8  "PTC GearboxIn11 Trq_out"
  Demux/7 -> BusCreator/7  "PTC GearboxIn11 Trq_in"
  Demux/6 -> BusCreator/6  "PTC GearboxIn11 rotv_out"
  Demux/5 -> BusCreator/5  "PTC GearboxIn11 rotv_in"
  Demux/4 -> BusCreator/4  "PTC GearboxIn11 i"
  Demux/3 -> BusCreator/3  "PTC GearboxIn11 Trq_DriveSrc_trg"
  Demux/2 -> BusCreator/2  "PTC GearboxIn11 GearNo_dis"
  Demux/1 -> BusCreator/1  "PTC GearboxIn11 GearNo"
  BusCreator/1 -> Out/1
  In/1 -> Demux/1

== system generic_src/CarMaker/IPG Vehicle/PowerTrain/PTControl Example/PTControl_In/CreateBus PTC GearboxIn2 ==
  In : Inport
  BusCreator : BusCreator  Inputs=20
  Demux : Demux  Outputs=20
      settings: DisplayOption=none
  Out : Outport  VectorParamsAs1DForOutWhenUnconnected=off
  wires:
  Demux/20 -> BusCreator/20  "PTC GearboxIn2 Clutch_dis i_TrqIn2Out"
  Demux/19 -> BusCreator/19  "PTC GearboxIn2 Clutch_dis Trq_out"
  Demux/18 -> BusCreator/18  "PTC GearboxIn2 Clutch_dis Trq_in"
  Demux/17 -> BusCreator/17  "PTC GearboxIn2 Clutch_dis rotv_out"
  Demux/16 -> BusCreator/16  "PTC GearboxIn2 Clutch_dis rotv_in"
  Demux/15 -> BusCreator/15  "PTC GearboxIn2 Clutch_dis Pos"
  Demux/14 -> BusCreator/14  "PTC GearboxIn2 Clutch i_TrqIn2Out"
  Demux/13 -> BusCreator/13  "PTC GearboxIn2 Clutch Trq_out"
  Demux/12 -> BusCreator/12  "PTC GearboxIn2 Clutch Trq_in"
  Demux/11 -> BusCreator/11  "PTC GearbxIn2 Clutch rotv_out"
  Demux/10 -> BusCreator/10  "PTC GearboxIn2 Clutch rotv_in"
  Demux/9 -> BusCreator/9  "PTC GearboxIn2 Clutch Pos"
  Demux/8 -> BusCreator/8  "PTC GearboxIn2 Trq_out"
  Demux/7 -> BusCreator/7  "PTC GearboxIn2 Trq_in"
  Demux/6 -> BusCreator/6  "PTC GearboxIn2 rotv_out"
  Demux/5 -> BusCreator/5  "PTC GearboxIn2 rotv_in"
  Demux/4 -> BusCreator/4  "PTC GearboxIn2 i"
  Demux/3 -> BusCreator/3  "PTC GearboxIn2 Trq_DriveSrc_trg"
  Demux/2 -> BusCreator/2  "PTC GearboxIn2 GearNo_dis"
  Demux/1 -> BusCreator/1  "PTC GearboxIn2 GearNo"
  BusCreator/1 -> Out/1
  In/1 -> Demux/1

== system generic_src/CarMaker/IPG Vehicle/PowerTrain/PTControl Example/PTControl_In/CreateBus PTC GearboxIn3 ==
  In : Inport
  BusCreator : BusCreator  Inputs=20
  Demux : Demux  Outputs=20
      settings: DisplayOption=none
  Out : Outport  VectorParamsAs1DForOutWhenUnconnected=off
  wires:
  Demux/20 -> BusCreator/20  "PTC GearboxIn3 Clutch_dis i_TrqIn2Out"
  Demux/19 -> BusCreator/19  "PTC GearboxIn3 Clutch_dis Trq_out"
  Demux/18 -> BusCreator/18  "PTC GearboxIn3 Clutch_dis Trq_in"
  Demux/17 -> BusCreator/17  "PTC GearboxIn3 Clutch_dis rotv_out"
  Demux/16 -> BusCreator/16  "PTC GearboxIn3 Clutch_dis rotv_in"
  Demux/15 -> BusCreator/15  "PTC GearboxIn3 Clutch_dis Pos"
  Demux/14 -> BusCreator/14  "PTC GearboxIn3 Clutch i_TrqIn2Out"
  Demux/13 -> BusCreator/13  "PTC GearboxIn3 Clutch Trq_out"
  Demux/12 -> BusCreator/12  "PTC GearboxIn3 Clutch Trq_in"
  Demux/11 -> BusCreator/11  "PTC GearboxIn3 Clutch rotv_out"
  Demux/10 -> BusCreator/10  "PTC GearboxIn3 Clutch rotv_in"
  Demux/9 -> BusCreator/9  "PTC GearboxIn3 Clutch Pos"
  Demux/8 -> BusCreator/8  "PTC GearboxIn3 Trq_out"
  Demux/7 -> BusCreator/7  "PTC GearboxIn3 Trq_in"
  Demux/6 -> BusCreator/6  "PTC GearboxIn3 rotv_out"
  Demux/5 -> BusCreator/5  "PTC GearboxIn3 rotv_in"
  Demux/4 -> BusCreator/4  "PTC GearboxIn3 i"
  Demux/3 -> BusCreator/3  "PTC GearboxIn3 Trq_DriveSrc_trg"
  Demux/2 -> BusCreator/2  "PTC GearboxIn3 GearNo_dis"
  Demux/1 -> BusCreator/1  "PTC GearboxIn3 GearNo"
  BusCreator/1 -> Out/1
  In/1 -> Demux/1

== system generic_src/CarMaker/IPG Vehicle/PowerTrain/PTControl Example/PTControl_In/CreateBus PTC GearboxIn4 ==
  In : Inport
  BusCreator : BusCreator  Inputs=20
  Demux : Demux  Outputs=20
      settings: DisplayOption=none
  Out : Outport  VectorParamsAs1DForOutWhenUnconnected=off
  wires:
  Demux/20 -> BusCreator/20  "PTC GearboxIn4 Clutch_dis i_TrqIn2Out"
  Demux/19 -> BusCreator/19  "PTC GearboxIn4 Clutch_dis Trq_out"
  Demux/18 -> BusCreator/18  "PTC GearboxIn4 Clutch_dis Trq_in"
  Demux/17 -> BusCreator/17  "PTC GearboxIn4 Clutch_dis rotv_out"
  Demux/16 -> BusCreator/16  "PTC GearboxIn4 Clutch_dis rotv_in"
  Demux/15 -> BusCreator/15  "PTC GearboxIn4 Clutch_dis Pos"
  Demux/14 -> BusCreator/14  "PTC GearboxIn4 Clutch i_TrqIn2Out"
  Demux/13 -> BusCreator/13  "PTC GearboxIn4 Clutch Trq_out"
  Demux/12 -> BusCreator/12  "PTC GearboxIn4 Clutch Trq_in"
  Demux/11 -> BusCreator/11  "PTC GearboxIn4 Clutch rotv_out"
  Demux/10 -> BusCreator/10  "PTC GearboxIn4 Clutch rotv_in"
  Demux/9 -> BusCreator/9  "PTC GearboxIn4 Clutch Pos"
  Demux/8 -> BusCreator/8  "PTC GearboxIn4 Trq_out"
  Demux/7 -> BusCreator/7  "PTC GearboxIn4 Trq_in"
  Demux/6 -> BusCreator/6  "PTC GearboxIn4 rotv_out"
  Demux/5 -> BusCreator/5  "PTC GearboxIn4 rotv_in"
  Demux/4 -> BusCreator/4  "PTC GearboxIn4 i"
  Demux/3 -> BusCreator/3  "PTC GearboxIn4 Trq_DriveSrc_trg"
  Demux/2 -> BusCreator/2  "PTC GearboxIn4 GearNo_dis"
  Demux/1 -> BusCreator/1  "PTC GearboxIn4 GearNo"
  BusCreator/1 -> Out/1
  In/1 -> Demux/1
